simulink model "mloc_statemachine"  (R2018b)
settings: configuration reference "Active" (kept outside this file)
settings Model: DataDictionary=mloc_statemachine.sldd  Creator=wischnewski  LastModifiedBy=ge34qer

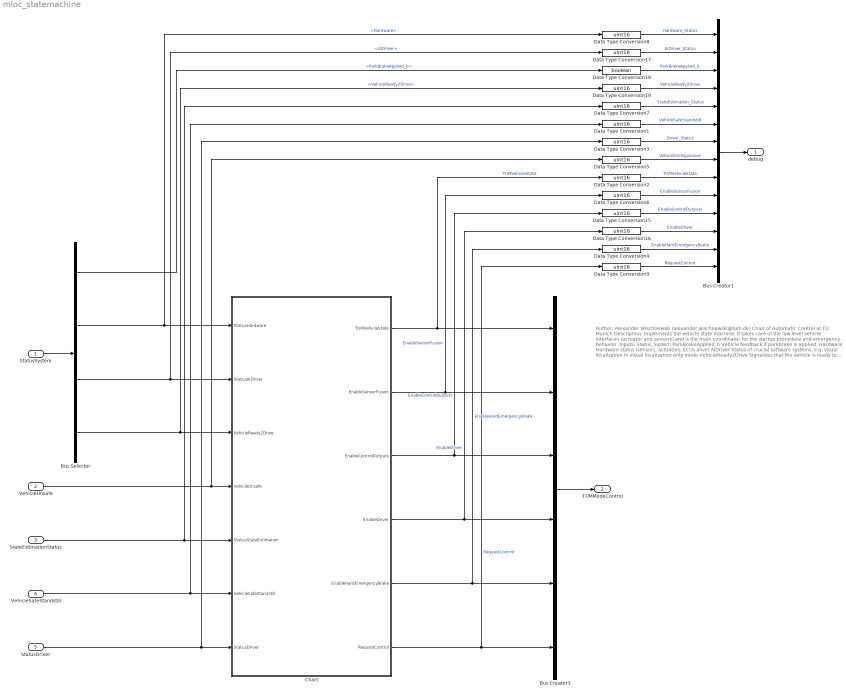
== system mloc_statemachine ==
  note: Author: Alexander Wischnewski (alexander.wischnewski@tum.de)
      | Chair of Automatic Control at TU Munich
      |
      | Description: Implements the vehicle state machine. It takes care of the low level vehicle interfaces (actuator and sensors)
      | and is the main coordinator for the startup procedure and emergency behavior.
      |
      | Inputs:
      | Status_System
      | ParkBrakeApplied_b Vehicle feedback if parkbrake is applied.
      | Hardware Hardware status (sensors, actuators, ECUs alive)
      | AIDriver Status of crucial software systems, e.g. visual localization in visual localization only mode
      | VehicleReady2Drive Signalizes that the vehicle is ready to drive and control is given to the software
      | (e.g. dead man switches are actuated)
      |
      | VehicleUnsafe Safety critical failure was detected
      | StateEstimationValid The fused vehicle state is ok
      | VehicleSafeStandstill The vehicle is in locked safe standstill position
      | DriverStatus The trajectory tracking driver status
      |
      | Outputs:
      | debug Debug information
      | TUMModeControl Control bits to interface the rest of the ECU software
  StatusSystem : Inport  OutDataTypeStr=Bus: VehicleSystemStatus
  VehicleUnsafe : Inport  Port=2  OutDataTypeStr=boolean
  StateEstimationStatus : Inport  Port=3  OutDataTypeStr=Enum: TUMHealthStatus
  VehicleSafeStandstill : Inport  Port=4  OutDataTypeStr=boolean
  StatusDriver : Inport  Port=5  OutDataTypeStr=Enum: TUMHealthStatus
  Bus Creator1 : BusCreator  Inputs=14  OutDataTypeStr=Bus: mloc_statemachine_debug
      settings: InheritFromInputs=off
  Bus Creator3 : BusCreator  Inputs=6
  Bus Selector : BusSelector  OutputSignals=ParkBrakeApplied_b,Hardware,AIDriver,VehicleReady2Drive
  Chart : Stateflow chart  TreatAsAtomicUnit=on
  Data Type Conversion{1..9,15..17,19} (13 alike) : DataTypeConversion  OutDataTypeStr=uint16
  Data Type Conversion18 : DataTypeConversion  OutDataTypeStr=boolean
  debug : Outport  OutDataTypeStr=Bus: mloc_statemachine_debug  BusOutputAsStruct=on
  TUMModeControl : Outport  Port=2  OutDataTypeStr=Bus: TUMModeControl  BusOutputAsStruct=on
  wires:
  Bus Selector/2 -> Data Type Conversion8/1, Chart/1(StatusHardware)  "<Hardware>"
  Data Type Conversion7/1 -> Bus Creator1/5  "StateEstimation_Status"
  Bus Creator1/1 -> debug/1
  VehicleUnsafe/1 -> Chart/4(VehicleUnsafe), Data Type Conversion5/1
  Data Type Conversion2/1 -> Bus Creator1/9  "TUMVehicleState"
  Data Type Conversion8/1 -> Bus Creator1/1  "Hardware_Status"
  StateEstimationStatus/1 -> Chart/5(StatusStateEstimation), Data Type Conversion7/1
  Bus Creator3/1 -> TUMModeControl/1
  VehicleSafeStandstill/1 -> Chart/6(VehicleSafeStandstill), Data Type Conversion1/1
  Chart/3(EnableControlOutputs) -> Bus Creator3/3, Data Type Conversion15/1  "EnableControlOutputs"
  StatusDriver/1 -> Chart/7(StatusDriver), Data Type Conversion3/1
  Chart/2(EnableSensorFusion) -> Bus Creator3/2, Data Type Conversion6/1  "EnableSensorFusion"
  Chart/1(TUMVehicleState) -> Bus Creator3/1, Data Type Conversion2/1  "TUMVehicleState"
  Chart/4(EnableDriver) -> Bus Creator3/4, Data Type Conversion16/1  "EnableDriver"
  Data Type Conversion1/1 -> Bus Creator1/6  "VehicleSafeStandstill"
  Data Type Conversion3/1 -> Bus Creator1/7  "Driver_Status"
  Data Type Conversion5/1 -> Bus Creator1/8  "VehicleUnresponsive"
  Data Type Conversion6/1 -> Bus Creator1/10  "EnableSensorFusion"
  Data Type Conversion15/1 -> Bus Creator1/11  "EnableControlOutputs"
  Data Type Conversion16/1 -> Bus Creator1/12  "EnableDriver"
  Chart/5(EnableHardEmergencyBrake) -> Data Type Conversion4/1, Bus Creator3/5  "EnableHardEmergencyBrake"
  Bus Selector/3 -> Data Type Conversion17/1, Chart/2(StatusAIDriver)  "<AIDriver>"
  Data Type Conversion19/1 -> Bus Creator1/4  "VehicleReady2Drive"
  Data Type Conversion18/1 -> Bus Creator1/3  "ParkBrakeApplied_b"
  Data Type Conversion17/1 -> Bus Creator1/2  "AIDriver_Status"
  Bus Selector/1 -> Data Type Conversion18/1  "<ParkBrakeApplied_b>"
  Chart/6(RequestControl) -> Data Type Conversion9/1, Bus Creator3/6  "RequestControl"
  StatusSystem/1 -> Bus Selector/1
  Bus Selector/4 -> Chart/3(VehicleReady2Drive), Data Type Conversion19/1  "<VehicleReady2Drive>"
  Data Type Conversion4/1 -> Bus Creator1/13  "EnableHardEmergencyBrake"
  Data Type Conversion9/1 -> Bus Creator1/14  "RequestControl"

== stateflow chart mloc_statemachine/Chart ==
  note: In general, the module mloc_statemachine is concerned with the vehicle side state handling.
      | This includes all vehicle sensors (acceleration, turn rates, vehicle speed, GPS, etc.) directly connected and used
      | by the vehicle controller. It is therefore not in charge of handling the communication with other parts of the software stack.
      | This task is done by the trajectory driver component. The reason for this distinction lies within the fact, that the vehicle
      | should be capable of using different "drivers", which may result in different functionality.
      |
      | The state machine can be roughly parted into three sections:
      | Startup: is present until all vehicle sensors and localization systems are ready
      | Idle: indicates that the basic vehicle functionality is available and the software
      | starts preparing communication with the rest of the software stack
      | ControlActive : hands over control to the trajectory tracking controller (trajectory driver) and handles emergency behavior
  state STARTUP
    entry:
    EnableDriver = false;
    EnableSensorFusion = false;
    state InitSG
      entry: TUMVehicleState = ...
      TUMVehicleState.STARTUP_Init;
    state WaitForSystem
      entry: TUMVehicleState = ...
      TUMVehicleState.STARTUP_WaitForSystem;
    state WaitForDriverComms
      entry: TUMVehicleState = ...
      TUMVehicleState.STARTUP_WaitForAIDriverComms;
    (junction 400) -> WaitForSystem [order 2]
    (junction 400) -> WaitForDriverComms [order 1] : [StatusHardware == OK]
    (default) -> InitSG
    WaitForSystem -> WaitForDriverComms : [StatusHardware == OK]
    InitSG -> WaitForSystem : after(2, sec)
    WaitForDriverComms -> WaitForSystem [order 2] : [StatusHardware ~= OK]
  state IDLE
    state SensorFusionReady
      state ActivateDriver
        entry:
        EnableDriver = true;
        RequestControl = false;
        TUMVehicleState = ...
        TUMVehicleState.IDLE_ActivateDriver;
      state WaitForDriver
        entry:
        TUMVehicleState = ...
        TUMVehicleState.IDLE_WaitForDriver;
      state WaitForVehicle
        entry: RequestControl = true;
        TUMVehicleState = ...
        TUMVehicleState.IDLE_WaitForVehicle;
      ActivateDriver -> WaitForDriver : after(1, sec)
      WaitForDriver -> WaitForVehicle : [StatusDriver == TUMHealthStatus.OK]
      (default) -> ActivateDriver
      WaitForVehicle -> ActivateDriver [order 2] : [StatusDriver ~= TUMHealthStatus.OK]
    state ActivateSensorFusion
      entry: TUMVehicleState = ...
      TUMVehicleState.IDLE_WaitForSensorFusion;
      EnableSensorFusion = true;
      EnableDriver = false;
    (default) -> ActivateSensorFusion
    ActivateSensorFusion -> SensorFusionReady : [after(3, sec) &&...
        |  StatusStateEstimation == TUMHealthStatus.OK]
    SensorFusionReady -> ActivateSensorFusion : [~(StatusStateEstimation == TUMHealthStatus.OK)]
  state ControlActive
    entry: EnableControlOutputs = true;
    exit: EnableControlOutputs = false;
    state NormalOperation
      state Driving
        entry:
        TUMVehicleState = ...
        TUMVehicleState.DRIVING;
      state SoftEmergencyStop
        entry:
        TUMVehicleState = ...
        TUMVehicleState.EMERGENCY;
      Driving -> SoftEmergencyStop : [~VehicleReady2Drive...
          | || StatusDriver == TUMHealthStatus.WARNING...
          | || StatusStateEstimation == TUMHealthStatus.WARNING...
          | || StatusAIDriver ~= OK]
    state HardEmergencyStop
      entry:
      TUMVehicleState = ...
      TUMVehicleState.HARDEMERGENCY;
      EnableHardEmergencyBrake = true;
    state Error
      entry:  EnableDriver = false;
    NormalOperation -> HardEmergencyStop : [StatusHardware ~= OK ||...
        | StatusDriver == TUMHealthStatus.ERROR ||...
        | StatusStateEstimation == TUMHealthStatus.ERROR || ...
        | VehicleUnsafe]
    HardEmergencyStop -> Error : [VehicleSafeStandstill]
    SoftEmergencyStop -> Error [order 1] : [VehicleSafeStandstill]
    SoftEmergencyStop -> HardEmergencyStop [order 2] : [after(P_VDC_SoftEmergencyTimeout_s, sec)]
  (default) -> STARTUP
  IDLE -> (junction 400) : [StatusHardware ~= OK...
      |  || StatusAIDriver ~= OK]
  WaitForDriverComms -> IDLE [order 1] : [StatusAIDriver == OK]
  WaitForVehicle -> Driving [order 1] : [VehicleReady2Drive &&...
      | VehicleSafeStandstill]
  data: StatusHardware input Enum: TUMHealthStatus; StatusAIDriver input Enum: TUMHealthStatus; VehicleReady2Drive input boolean; TUMVehicleState output Enum: TUMVehicleState =TUMVehicleState.OFF; VehicleUnsafe input boolean; StatusStateEstimation input Enum: TUMHealthStatus; EnableSensorFusion output boolean =false; VehicleSafeStandstill input boolean; EnableControlOutputs output boolean =false; StatusDriver input Enum: TUMHealthStatus; EnableDriver output boolean =false; EnableHardEmergencyBrake output boolean =false; P_VDC_SoftEmergencyTimeout_s parameter; RequestControl output boolean
